simulink model "test_PLECS"  (R2023b)
settings: Solver=VariableStepAuto  StartTime=0.0  StopTime=0.0117  FixedStep=6.5e-6  MaxStep=6.5e-6  MinStep=4.5e-6  RelTol=1e-3
undefined symbols (not defined in the file or in its folder): plecs
libraries: simulink_extras x8
settings Model: Creator=Nelson  LastModifiedBy=franc

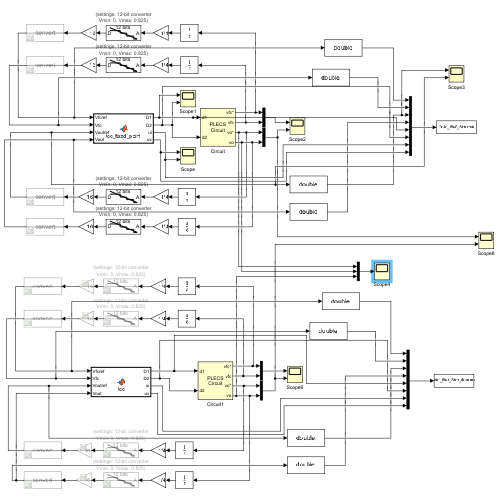
[thumbnail: Simulink's stored preview of the top-level diagram]
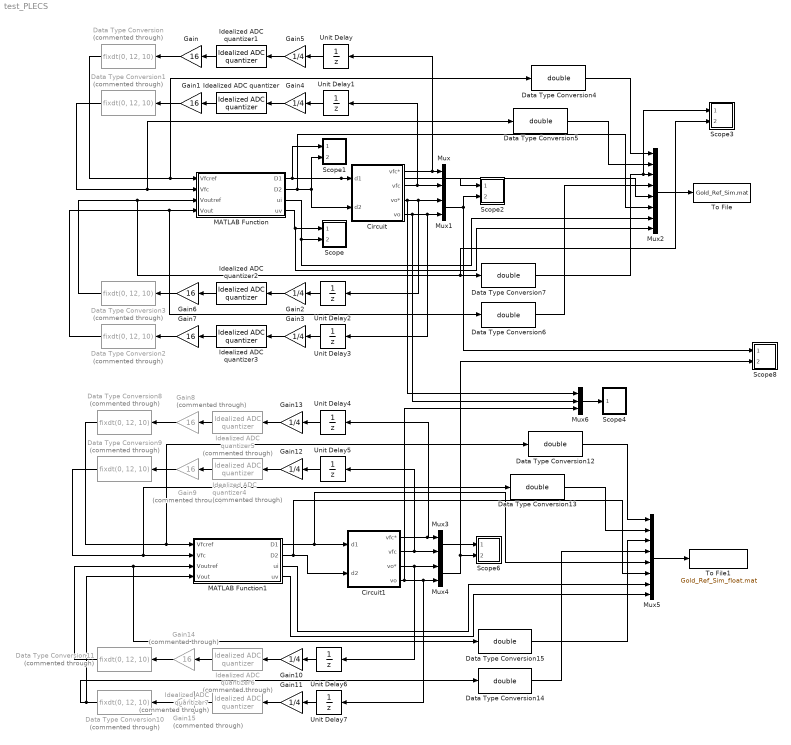
== system test_PLECS ==
  Circuit : Subsystem  LoadFcn=plecs('sl', 200);  InitFcn=plecs('sl', 214);  StartFcn=plecs('sl', 208);  StopFcn=plecs('sl', 209);  mask(PlecsCircuit){PLECSData=<binary blob, 9000 chars, not shown>}
      mask prompts: PLECSData "PLECS Data (Do not delete or modify!)"
      mask init:
      | % PLACE CUSTOM INITIALIZATIONS ABOVE
      | % DO NOT REMOVE
      | plecs('sl', 215);
      | % DO NOT REMOVE
      settings: CopyFcn=plecs('sl', 203);  DeleteFcn=plecs('sl', 205);  UndoDeleteFcn=plecs('sl', 206);  PreSaveFcn=plecs('sl', 211);  PostSaveFcn=plecs('sl', 201);  NameChangeFcn=plecs('sl', 210);  DestroyFcn=plecs('sl', 207);  PreCopyFcn=plecs('sl', 216);  OpenFcn=plecs('sl', 202);  ErrorFcn=plerrorfcn
      mask Help: eval('plecs(''help'', ''qthelp:///creatingacircuit.html'')')
      mask Display: disp('PLECS\nCircuit')
  Circuit1 : Subsystem  LoadFcn=plecs('sl', 200);  InitFcn=plecs('sl', 214);  StartFcn=plecs('sl', 208);  StopFcn=plecs('sl', 209);  mask(PlecsCircuit){PLECSData=<binary blob, 8936 chars, not shown>}
      mask prompts: PLECSData "PLECS Data (Do not delete or modify!)"
      mask init:
      | % PLACE CUSTOM INITIALIZATIONS ABOVE
      | % DO NOT REMOVE
      | plecs('sl', 215);
      | % DO NOT REMOVE
      settings: CopyFcn=plecs('sl', 203);  DeleteFcn=plecs('sl', 205);  UndoDeleteFcn=plecs('sl', 206);  PreSaveFcn=plecs('sl', 211);  PostSaveFcn=plecs('sl', 201);  NameChangeFcn=plecs('sl', 210);  DestroyFcn=plecs('sl', 207);  PreCopyFcn=plecs('sl', 216);  OpenFcn=plecs('sl', 202);  ErrorFcn=plerrorfcn
      mask Help: eval('plecs(''help'', ''qthelp:///creatingacircuit.html'')')
      mask Display: disp('PLECS\nCircuit')
  Data Type Conversion{,1..3,8..11} (8 alike) : DataTypeConversion  Commented=through  OutDataTypeStr=fixdt(0, 12, 10)  RndMeth=Nearest
  Data Type Conversion{4..7,12..15} (8 alike) : DataTypeConversion  OutDataTypeStr=double  RndMeth=Nearest
  Gain{,1,6..7} (4 alike) : Gain  Gain=16  OutDataTypeStr=uint16  RndMeth=Nearest  SaturateOnIntegerOverflow=on
  Gain{2..5,10..13} (8 alike) : Gain  Gain=1/4
  Gain{8..9,14..15} (4 alike) : Gain  Commented=through  Gain=16  OutDataTypeStr=uint16  RndMeth=Nearest  SaturateOnIntegerOverflow=on
  Idealized ADC quantizer{,1..3} (4 alike) : simulink_extras/Additional Discrete/Idealized ADC quantizer  NumberOfConverterBits=12  Vmin=0  Vmax=0.825  OutputDataType=uint16  OutputNegativeValues=off
  Idealized ADC quantizer4 : simulink_extras/Additional Discrete/Idealized ADC quantizer  Commented=through  NumberOfConverterBits=12  Vmin=0  Vmax=0.825  OutputDataType=double  OutputNegativeValues=off
  Idealized ADC quantizer5 : simulink_extras/Additional Discrete/Idealized ADC quantizer  Commented=through  NumberOfConverterBits=12  Vmin=0  Vmax=0.825  OutputDataType=double  OutputNegativeValues=off
  Idealized ADC quantizer6 : simulink_extras/Additional Discrete/Idealized ADC quantizer  Commented=through  NumberOfConverterBits=12  Vmin=0  Vmax=0.825  OutputDataType=uint16  OutputNegativeValues=off
  Idealized ADC quantizer7 : simulink_extras/Additional Discrete/Idealized ADC quantizer  Commented=through  NumberOfConverterBits=12  Vmin=0  Vmax=0.825  OutputDataType=uint16  OutputNegativeValues=off
  MATLAB Function : MATLAB Function  TreatAsAtomicUnit=on
  MATLAB Function1 : MATLAB Function  TreatAsAtomicUnit=on
  Mux{,1,3..4} (4 alike) : Mux  Inputs=2
  Mux2 : Mux  Inputs=8
  Mux5 : Mux  Inputs=8
  Mux6 : Mux  Inputs=3
  Scope : Subsystem  LoadFcn=plecs('sl', 300);  InitFcn=plecs('sl', 314);  StartFcn=plecs('sl', 308);  StopFcn=plecs('sl', 309);  mask{Settings=<binary blob, 900 chars, not shown>}
      mask init:
      | plecs('sl', 315);
      settings: CopyFcn=plecs('sl', 303);  DeleteFcn=plecs('sl', 305);  UndoDeleteFcn=plecs('sl', 306);  PreSaveFcn=plecs('sl', 311);  NameChangeFcn=plecs('sl', 310);  DestroyFcn=plecs('sl', 307);  OpenFcn=plecs('sl', 302);  ErrorFcn=plerrorfcn
      mask Display: plot([0.1 0.9 0.9 0.1 0.1], [0.9 0.9 0.5 0.5 0.9])
  Scope1 : Subsystem  LoadFcn=plecs('sl', 300);  InitFcn=plecs('sl', 314);  StartFcn=plecs('sl', 308);  StopFcn=plecs('sl', 309);  mask{Settings=<binary blob, 888 chars, not shown>}
      mask init:
      | plecs('sl', 315);
      settings: CopyFcn=plecs('sl', 303);  DeleteFcn=plecs('sl', 305);  UndoDeleteFcn=plecs('sl', 306);  PreSaveFcn=plecs('sl', 311);  NameChangeFcn=plecs('sl', 310);  DestroyFcn=plecs('sl', 307);  OpenFcn=plecs('sl', 302);  ErrorFcn=plerrorfcn
      mask Display: plot([0.1 0.9 0.9 0.1 0.1], [0.9 0.9 0.5 0.5 0.9])
  Scope2 : Subsystem  LoadFcn=plecs('sl', 300);  InitFcn=plecs('sl', 314);  StartFcn=plecs('sl', 308);  StopFcn=plecs('sl', 309);  mask{Settings=<binary blob, 1240 chars, not shown>}
      mask init:
      | plecs('sl', 315);
      settings: CopyFcn=plecs('sl', 303);  DeleteFcn=plecs('sl', 305);  UndoDeleteFcn=plecs('sl', 306);  PreSaveFcn=plecs('sl', 311);  NameChangeFcn=plecs('sl', 310);  DestroyFcn=plecs('sl', 307);  OpenFcn=plecs('sl', 302);  ErrorFcn=plerrorfcn
      mask Display: plot([0.1 0.9 0.9 0.1 0.1], [0.9 0.9 0.5 0.5 0.9])
  Scope3 : Subsystem  LoadFcn=plecs('sl', 300);  InitFcn=plecs('sl', 314);  StartFcn=plecs('sl', 308);  StopFcn=plecs('sl', 309);  mask{Settings=<binary blob, 1240 chars, not shown>}
      mask init:
      | plecs('sl', 315);
      settings: CopyFcn=plecs('sl', 303);  DeleteFcn=plecs('sl', 305);  UndoDeleteFcn=plecs('sl', 306);  PreSaveFcn=plecs('sl', 311);  NameChangeFcn=plecs('sl', 310);  DestroyFcn=plecs('sl', 307);  OpenFcn=plecs('sl', 302);  ErrorFcn=plerrorfcn
      mask Display: plot([0.1 0.9 0.9 0.1 0.1], [0.9 0.9 0.5 0.5 0.9])
  Scope4 : Subsystem  LoadFcn=plecs('sl', 300);  InitFcn=plecs('sl', 314);  StartFcn=plecs('sl', 308);  StopFcn=plecs('sl', 309);  mask{Settings=<binary blob, 968 chars, not shown>}
      mask init:
      | plecs('sl', 315);
      settings: CopyFcn=plecs('sl', 303);  DeleteFcn=plecs('sl', 305);  UndoDeleteFcn=plecs('sl', 306);  PreSaveFcn=plecs('sl', 311);  NameChangeFcn=plecs('sl', 310);  DestroyFcn=plecs('sl', 307);  OpenFcn=plecs('sl', 302);  ErrorFcn=plerrorfcn
      mask Display: plot([0.1 0.9 0.9 0.1 0.1], [0.9 0.9 0.5 0.5 0.9])
  Scope6 : Subsystem  LoadFcn=plecs('sl', 300);  InitFcn=plecs('sl', 314);  StartFcn=plecs('sl', 308);  StopFcn=plecs('sl', 309);  mask{Settings=<binary blob, 1240 chars, not shown>}
      mask init:
      | plecs('sl', 315);
      settings: CopyFcn=plecs('sl', 303);  DeleteFcn=plecs('sl', 305);  UndoDeleteFcn=plecs('sl', 306);  PreSaveFcn=plecs('sl', 311);  NameChangeFcn=plecs('sl', 310);  DestroyFcn=plecs('sl', 307);  OpenFcn=plecs('sl', 302);  ErrorFcn=plerrorfcn
      mask Display: plot([0.1 0.9 0.9 0.1 0.1], [0.9 0.9 0.5 0.5 0.9])
  Scope8 : Subsystem  LoadFcn=plecs('sl', 300);  InitFcn=plecs('sl', 314);  StartFcn=plecs('sl', 308);  StopFcn=plecs('sl', 309);  mask{Settings=<binary blob, 1196 chars, not shown>}
      mask init:
      | plecs('sl', 315);
      settings: CopyFcn=plecs('sl', 303);  DeleteFcn=plecs('sl', 305);  UndoDeleteFcn=plecs('sl', 306);  PreSaveFcn=plecs('sl', 311);  NameChangeFcn=plecs('sl', 310);  DestroyFcn=plecs('sl', 307);  OpenFcn=plecs('sl', 302);  ErrorFcn=plerrorfcn
      mask Display: plot([0.1 0.9 0.9 0.1 0.1], [0.9 0.9 0.5 0.5 0.9])
  To File : ToFile  Filename=Gold_Ref_Sim.mat  SampleTime=6.5e-6
  To File1 : ToFile  Filename=Gold_Ref_Sim_float.mat  SampleTime=6.5e-6
  Unit Delay{,1..7} (8 alike) : UnitDelay  SampleTime=-1  HasFrameUpgradeWarning=on
  wires:
  MATLAB Function/2(D2) -> Mux2/6, Scope1/2(2), Circuit/2(d2)
  MATLAB Function/4(uv) -> Mux2/8, Scope/1(1)
  MATLAB Function/3(ui) -> Mux2/7, Scope/2(2)
  Circuit/1(vfc*) -> Unit Delay/1, Mux/1
  Circuit/2(vfc) -> Unit Delay1/1, Mux/2
  Circuit/3(vo*) -> Mux6/1, Unit Delay2/1, Mux1/1
  Circuit/4(vo) -> Mux6/2, Unit Delay3/1, Mux1/2
  Mux/1 -> Scope2/1(1)
  Mux1/1 -> Scope2/2(2), Scope8/1(1)
  Unit Delay2/1 -> Gain2/1
  Idealized ADC quantizer1/1 -> Gain/1
  Gain/1 -> Data Type Conversion/1
  Idealized ADC quantizer/1 -> Gain1/1
  Data Type Conversion/1 -> Data Type Conversion4/1, MATLAB Function/1(Vfcref)
  Gain1/1 -> Data Type Conversion1/1
  Data Type Conversion1/1 -> Data Type Conversion5/1, MATLAB Function/2(Vfc)
  Idealized ADC quantizer3/1 -> Gain7/1
  Idealized ADC quantizer2/1 -> Gain6/1
  Data Type Conversion3/1 -> Scope3/2(2), Data Type Conversion7/1, MATLAB Function/3(Voutref)
  Gain2/1 -> Idealized ADC quantizer2/1
  Unit Delay3/1 -> Gain3/1
  Gain3/1 -> Idealized ADC quantizer3/1
  Gain4/1 -> Idealized ADC quantizer/1
  Unit Delay1/1 -> Gain4/1
  Gain5/1 -> Idealized ADC quantizer1/1
  Unit Delay/1 -> Gain5/1
  Gain6/1 -> Data Type Conversion3/1
  Gain7/1 -> Data Type Conversion2/1
  Mux2/1 -> To File/1
  Data Type Conversion4/1 -> Mux2/1
  Data Type Conversion5/1 -> Mux2/2
  Data Type Conversion2/1 -> Data Type Conversion6/1, MATLAB Function/4(Vout)
  MATLAB Function/1(D1) -> Scope1/1(1), Mux2/5, Circuit/1(d1)
  Data Type Conversion6/1 -> Mux2/4
  Data Type Conversion7/1 -> Scope3/1(1), Mux2/3
  Data Type Conversion13/1 -> Mux5/2
  Gain15/1 -> Data Type Conversion10/1
  Mux5/1 -> To File1/1
  Data Type Conversion12/1 -> Mux5/1
  Unit Delay4/1 -> Gain13/1
  Data Type Conversion14/1 -> Mux5/4
  Gain14/1 -> Data Type Conversion11/1
  Idealized ADC quantizer4/1 -> Gain9/1
  Gain8/1 -> Data Type Conversion8/1
  Circuit1/1(vfc*) -> Unit Delay4/1, Mux3/1
  Data Type Conversion8/1 -> Data Type Conversion12/1, MATLAB Function1/1(Vfcref)
  Idealized ADC quantizer7/1 -> Gain15/1
  Mux4/1 -> Scope6/2(2), Scope8/2(2)
  Circuit1/3(vo*) -> Unit Delay6/1, Mux4/1
  Unit Delay5/1 -> Gain12/1
  Data Type Conversion11/1 -> Data Type Conversion15/1, MATLAB Function1/3(Voutref)
  Unit Delay7/1 -> Gain11/1
  Gain11/1 -> Idealized ADC quantizer7/1
  Gain9/1 -> Data Type Conversion9/1
  Gain13/1 -> Idealized ADC quantizer5/1
  Circuit1/4(vo) -> Mux6/3, Unit Delay7/1, Mux4/2
  Data Type Conversion9/1 -> Data Type Conversion13/1, MATLAB Function1/2(Vfc)
  MATLAB Function1/3(ui) -> Mux5/7
  Data Type Conversion10/1 -> Data Type Conversion14/1, MATLAB Function1/4(Vout)
  MATLAB Function1/1(D1) -> Circuit1/1(d1), Mux5/5
  Circuit1/2(vfc) -> Unit Delay5/1, Mux3/2
  Idealized ADC quantizer6/1 -> Gain14/1
  Gain10/1 -> Idealized ADC quantizer6/1
  MATLAB Function1/4(uv) -> Mux5/8
  MATLAB Function1/2(D2) -> Mux5/6, Circuit1/2(d2)
  Data Type Conversion15/1 -> Mux5/3
  Idealized ADC quantizer5/1 -> Gain8/1
  Unit Delay6/1 -> Gain10/1
  Gain12/1 -> Idealized ADC quantizer4/1
  Mux3/1 -> Scope6/1(1)
  Mux6/1 -> Scope4/1(1)

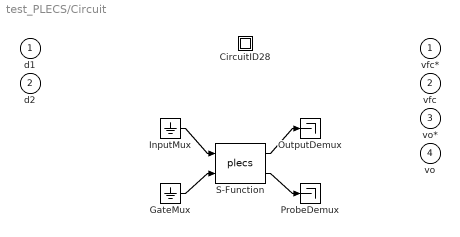
== system test_PLECS/Circuit ==
  d1 : Inport  PortDimensions=1
  d2 : Inport  Port=2  PortDimensions=1
  " CircuitID28 " : Subsystem
  " GateMux " : Ground
  " InputMux " : Ground
  " OutputDemux " : Terminator
  " ProbeDemux " : Terminator
  " S-Function " : S-Function  FunctionName=plecs  SFunctionDeploymentMode=off  EnableBusSupport=off
  vfc* : Outport  PortDimensions=1
  vfc : Outport  Port=2  PortDimensions=1
  vo* : Outport  Port=3  PortDimensions=1
  vo : Outport  Port=4  PortDimensions=1
  wires:
  " InputMux "/1 -> " S-Function "/1
  " GateMux "/1 -> " S-Function "/2
  " S-Function "/1 -> " OutputDemux "/1
  " S-Function "/2 -> " ProbeDemux "/1

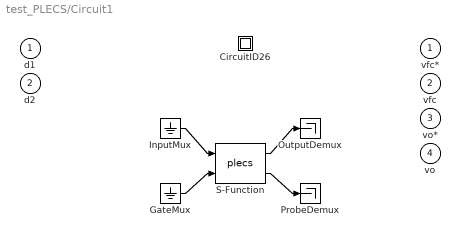
== system test_PLECS/Circuit1 ==
  d1 : Inport  PortDimensions=1
  d2 : Inport  Port=2  PortDimensions=1
  " CircuitID26 " : Subsystem
  " GateMux " : Ground
  " InputMux " : Ground
  " OutputDemux " : Terminator
  " ProbeDemux " : Terminator
  " S-Function " : S-Function  FunctionName=plecs  SFunctionDeploymentMode=off  EnableBusSupport=off
  vfc* : Outport  PortDimensions=1
  vfc : Outport  Port=2  PortDimensions=1
  vo* : Outport  Port=3  PortDimensions=1
  vo : Outport  Port=4  PortDimensions=1
  wires:
  " InputMux "/1 -> " S-Function "/1
  " GateMux "/1 -> " S-Function "/2
  " S-Function "/1 -> " OutputDemux "/1
  " S-Function "/2 -> " ProbeDemux "/1

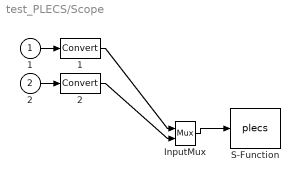
== system test_PLECS/Scope ==
  1 : Inport
  2 : Inport  Port=2
  " 1 " : DataTypeConversion
  " 2 " : DataTypeConversion
  " InputMux " : Mux  Inputs=2
  " S-Function " : S-Function  FunctionName=plecs  SFunctionDeploymentMode=off  EnableBusSupport=off
  wires:
  " InputMux "/1 -> " S-Function "/1
  1/1 -> " 1 "/1
  " 1 "/1 -> " InputMux "/1
  2/1 -> " 2 "/1
  " 2 "/1 -> " InputMux "/2

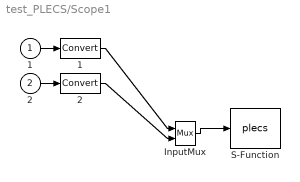
== system test_PLECS/Scope1 ==
  1 : Inport
  2 : Inport  Port=2
  " 1 " : DataTypeConversion
  " 2 " : DataTypeConversion
  " InputMux " : Mux  Inputs=2
  " S-Function " : S-Function  FunctionName=plecs  SFunctionDeploymentMode=off  EnableBusSupport=off
  wires:
  " InputMux "/1 -> " S-Function "/1
  1/1 -> " 1 "/1
  " 1 "/1 -> " InputMux "/1
  2/1 -> " 2 "/1
  " 2 "/1 -> " InputMux "/2

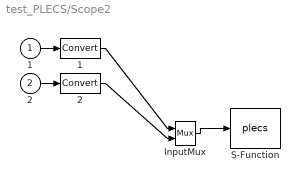
== system test_PLECS/Scope2 ==
  1 : Inport
  2 : Inport  Port=2
  " 1 " : DataTypeConversion
  " 2 " : DataTypeConversion
  " InputMux " : Mux  Inputs=2
  " S-Function " : S-Function  FunctionName=plecs  SFunctionDeploymentMode=off  EnableBusSupport=off
  wires:
  " InputMux "/1 -> " S-Function "/1
  1/1 -> " 1 "/1
  " 1 "/1 -> " InputMux "/1
  2/1 -> " 2 "/1
  " 2 "/1 -> " InputMux "/2

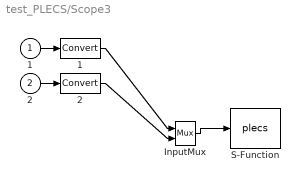
== system test_PLECS/Scope3 ==
  1 : Inport
  2 : Inport  Port=2
  " 1 " : DataTypeConversion
  " 2 " : DataTypeConversion
  " InputMux " : Mux  Inputs=2
  " S-Function " : S-Function  FunctionName=plecs  SFunctionDeploymentMode=off  EnableBusSupport=off
  wires:
  " InputMux "/1 -> " S-Function "/1
  1/1 -> " 1 "/1
  " 1 "/1 -> " InputMux "/1
  2/1 -> " 2 "/1
  " 2 "/1 -> " InputMux "/2

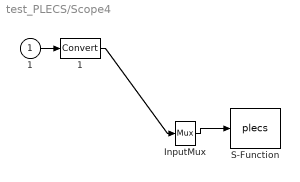
== system test_PLECS/Scope4 ==
  1 : Inport
  " 1 " : DataTypeConversion
  " InputMux " : Mux  Inputs=1
  " S-Function " : S-Function  FunctionName=plecs  SFunctionDeploymentMode=off  EnableBusSupport=off
  wires:
  " InputMux "/1 -> " S-Function "/1
  1/1 -> " 1 "/1
  " 1 "/1 -> " InputMux "/1

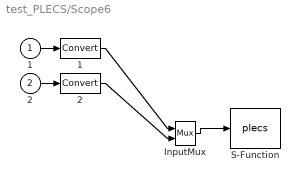
== system test_PLECS/Scope6 ==
  1 : Inport
  2 : Inport  Port=2
  " 1 " : DataTypeConversion
  " 2 " : DataTypeConversion
  " InputMux " : Mux  Inputs=2
  " S-Function " : S-Function  FunctionName=plecs  SFunctionDeploymentMode=off  EnableBusSupport=off
  wires:
  " InputMux "/1 -> " S-Function "/1
  1/1 -> " 1 "/1
  " 1 "/1 -> " InputMux "/1
  2/1 -> " 2 "/1
  " 2 "/1 -> " InputMux "/2

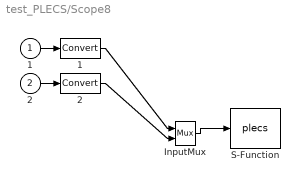
== system test_PLECS/Scope8 ==
  1 : Inport
  2 : Inport  Port=2
  " 1 " : DataTypeConversion
  " 2 " : DataTypeConversion
  " InputMux " : Mux  Inputs=2
  " S-Function " : S-Function  FunctionName=plecs  SFunctionDeploymentMode=off  EnableBusSupport=off
  wires:
  " InputMux "/1 -> " S-Function "/1
  1/1 -> " 1 "/1
  " 1 "/1 -> " InputMux "/1
  2/1 -> " 2 "/1
  " 2 "/1 -> " InputMux "/2

== system test_PLECS/Circuit/ CircuitID28  ==

== system test_PLECS/Circuit1/ CircuitID26  ==

== matlab function test_PLECS/MATLAB Function1 ==
  data: Vfcref input; Vfc input; Voutref input; Vout input; D1 output; D2 output; ui output; uv output
function [D1, D2, ui, uv] = fcc(Vfcref, Vfc, Voutref, Vout)
    % Kpv =  3.214624;
    % Kiv = -1.410335;
    % Kpc =  12.58407884;
    % Kic = -12.410690825;
    % MAX_DUTY_CYCLE = (127);
    % gain = 4/65535;
    % 
    % ui_aux = pivo_fun(Voutref*gain, Vout*gain, 0.0, 127.0, Kpv, Kiv);
    % uv_aux = pivf_fun(Vfcref*gain , Vfc*gain , -38.0, 38.0, Kpc, Kic);

    Kpv = 0.025312;
    Kiv = -0.011105;
    Kpc =  0.099087235;
    Kic = -0.097721975;
    MAX_DUTY_CYCLE = (127);
    gain = 4;

    ui_aux = pivo_fun(Voutref*gain, Vout*gain, 0.0, 1.0, Kpv, Kiv);
    uv_aux = pivf_fun(Vfcref*gain , Vfc*gain , -0.3, 0.3, Kpc, Kic);


    D1_aux = ((ui_aux) + (uv_aux))*MAX_DUTY_CYCLE;
    D2_aux = ((ui_aux) - (uv_aux))*MAX_DUTY_CYCLE;

    D1  = max(0, min(D1_aux, MAX_DUTY_CYCLE));
    D2  = max(0, min(D2_aux, MAX_DUTY_CYCLE));

    ui = (ui_aux);
    uv = (uv_aux);
end

%function out = pivf_fun(varargin)
function out = pivf_fun(Vrk, Vk, Vmin, Vmax, Kpid, Kiid)
    % Declarar todas las variables persistentes al inicio
    persistent Kp Ki KUi KXi
    persistent xVrk xVk xVmax xVmin xXik xUik xVmk

    % Inicializar si es primera vez
    if isempty(xXik)
        xXik = zeros(1, 2);
        xUik = zeros(1, 2);
    end

    % Asignación de parámetros
    xVrk = Vrk;
    xVk = Vk;
    xVmax = Vmax;
    xVmin = Vmin;
    Kp = Kpid;
    Ki = Kiid;
    KUi = -(Kp + Ki)/(Kp * Kpid);
    KXi = -Ki / Kp;

    % PI cálculo
    xXik(2) = xXik(1);
    xUik(2) = xUik(1);
    xXik(1) = KUi * xUik(2) + KXi * xXik(2);
    xUik(1) = Kp * (xVrk - xVk - xXik(1));
    xUik(1) = min(max(xUik(1), xVmin), xVmax);

    xVmk = xUik(1);
    out = xVmk;
end

%function out = pivf_fun(varargin)
function out = pivo_fun(Vrk, Vk, Vmin, Vmax, Kpid, Kiid)
    % Declarar todas las variables persistentes al inicio
    persistent Kp Ki KUi KXi
    persistent xVrk xVk xVmax xVmin xXik xUik xVmk

    % Inicializar si es primera vez
    if isempty(xXik)
        xXik = zeros(1, 2);
        xUik = zeros(1, 2);
    end

    % Asignación de parámetros
    xVrk = Vrk;
    xVk = Vk;
    xVmax = Vmax;
    xVmin = Vmin;
    Kp = Kpid;
    Ki = Kiid;
    KUi = -(Kp + Ki)/(Kp * Kpid);
    KXi = -Ki / Kp;

    % PI cálculo
    xXik(2) = xXik(1);
    xUik(2) = xUik(1);
    xXik(1) = KUi * xUik(2) + KXi * xXik(2);
    xUik(1) = Kp * (xVrk - xVk - xXik(1));
    xUik(1) = min(max(xUik(1), xVmin), xVmax);

    xVmk = xUik(1);
    out = xVmk;
end

== matlab function test_PLECS/MATLAB Function ==
  data: Vfcref input; Vfc input; Voutref input; Vout input; D1 output; D2 output; ui output; uv output
%%%%%%%%%%%%%%%%%%%%%%%%%%%%%%%%%%%%%%%%%%%%%%%%%%%%%%%%%%%%%%%%%%%%%%%%%%%%
%                                                                          %
%          Generated by MATLAB 23.2 and Fixed-Point Designer 23.2          %
%                                                                          %
%%%%%%%%%%%%%%%%%%%%%%%%%%%%%%%%%%%%%%%%%%%%%%%%%%%%%%%%%%%%%%%%%%%%%%%%%%%%
function [D1,D2,ui,uv] = fcc_fixed_point(Vfcref,Vfc,Voutref,Vout)
    fm = get_fimath();
    Vfcref_in = fi( Vfcref, 0, 16, 0, fm );
    Vfc_in = fi( Vfc, 0, 16, 0, fm );
    Voutref_in = fi( Voutref, 0, 16, 0, fm );
    Vout_in = fi( Vout, 0, 16, 0, fm );
    [D1_out,D2_out,ui_out,uv_out] = fcc_fixpt( Vfcref_in, Vfc_in, Voutref_in, Vout_in );
    D1 = double( D1_out );
    D2 = double( D2_out );
    ui = double( ui_out );
    uv = double( uv_out );
end

function [D1, D2, ui, uv] = fcc_fixpt(Vfcref, Vfc, Voutref, Vout)
    fm = get_fimath();

    Kpv =  fi(3.214624, 1, 22, 14, fm);
    Kiv = fi(-1.4105, 1, 22, 14, fm);fi(335, 0, 9, 0, fm);
    Kpc =  fi(12.58407884, 1, 22, 14, fm);
    Kic = fi(-12.410690825, 1, 22, 14, fm);
    MAX_DUTY_CYCLE = fi((127), 0, 8, 0, fm);
    gain = fi(4/65535, 1, 22, 14, fm);
    %D1_aux = int8(0);
    %D2_aux = int8(0);

    % Calculo de actuaciones desacopladas
    %ui_aux = int8(0);
    %uv_aux = int8(0);
    ui_aux = fi(pivo_fun(fi(Voutref*gain, 1, 22, 14, fm), fi(Vout*gain, 1, 22, 14, fm), fi(fi(0.0, 0, 1, 0, fm), 1, 22, 14, fm), fi(fi(127.0, 0, 7, 0, fm), 1, 22, 14, fm), fi(Kpv, 1, 22, 14, fm), fi(Kiv, 1, 22, 14, fm)), 1, 22, 14, fm);
    uv_aux = fi(pivf_fun(fi(Vfcref*gain, 1, 22, 14, fm) , fi(Vfc*gain, 1, 22, 14, fm) , fi(fi(-38.0, 1, 7, 0, fm), 1, 22, 14, fm), fi(fi(38.0, 0, 6, 0, fm), 1, 22, 14, fm), fi(Kpc, 1, 22, 14, fm), fi(Kic, 1, 22, 14, fm)), 1, 22, 14, fm);


    D1_aux = fi(fix((ui_aux) + (uv_aux)), 0, 8, 0, fm);
    D2_aux = fi(fix((ui_aux) - (uv_aux)), 0, 8, 0, fm);

    D1 = fi((min(D1_aux, MAX_DUTY_CYCLE)), 0, 8, 0, fm);
    D2 = fi((min(D2_aux, MAX_DUTY_CYCLE)), 0, 8, 0, fm);

    ui = fi((ui_aux), 0, 8, 0, fm);
    uv = fi((uv_aux), 0, 8, 0, fm);
end

%function out = pivf_fun(varargin)
function out = pivo_fun(Vrk, Vk, Vmin, Vmax, Kpid, Kiid)
    % Declarar todas las variables persistentes al inicio
    fm = get_fimath();

    persistent Kp Ki KUi KXi
    persistent xVrk xVk xVmax xVmin xXik xUik xVmk

    % --------------------------
    % Caso: RESET con un solo argumento
    % --------------------------
    %if nargin == 1 && islogical(varargin{1}) && varargin{1} == true
    %    clear pivo_fun
    %    out = 0.0;
    %    return
    %end

    % --------------------------
    % Caso: operación normal
    % --------------------------
    %if nargin ~= 7
    %    error('pivo_fun: Expected 7 input arguments or reset flag.');
    %end

    % Extraer argumentos normalmente
    %Vrk  = varargin{1};
    %Vk   = varargin{2};
    %Vmin = varargin{3};
    %Vmax = varargin{4};
    %Kpid = varargin{5};
    %Kiid = varargin{6};
    %reset = varargin{7}; %#ok<NASGU>  % No se usa ya

    % Inicializar si es primera vez
    if isempty(xXik)
        xXik = fi(zeros(1, 2), 1, 22, 14, fm);
        xUik = fi(zeros(1, 2), 1, 22, 14, fm);
    end

    % Asignación de parámetros
    xVrk = fi(Vrk, 1, 22, 14, fm);
    xVk = fi(Vk, 1, 22, 14, fm);
    xVmax = fi(Vmax, 1, 22, 14, fm);
    xVmin = fi(Vmin, 1, 22, 14, fm);
    Kp = fi(Kpid, 1, 22, 14, fm);
    Ki = fi(Kiid, 1, 22, 14, fm);
    KUi = fi(fi_div(fi_uminus((Kp + Ki)), (Kp * Kpid)), 1, 22, 14, fm);
    KXi = fi(fi_div(fi_uminus(Ki), Kp), 1, 22, 14, fm);

    % PI cálculo
    xXik(2) = xXik(1);
    xUik(2) = xUik(1);
    xXik(1) = KUi * xUik(2) + KXi * xXik(2);
    xUik(1) = Kp * (xVrk - xVk - xXik(1));
    xUik(1) = min(max(xUik(1), xVmin), xVmax);

    xVmk = fi(xUik(1), 1, 22, 14, fm);
    out = fi(xVmk, 1, 22, 14, fm);
end

%function out = pivf_fun(varargin)
function out = pivf_fun(Vrk, Vk, Vmin, Vmax, Kpid, Kiid)
    % Declarar todas las variables persistentes al inicio
    fm = get_fimath();

    persistent Kp Ki KUi KXi
    persistent xVrk xVk xVmax xVmin xXik xUik xVmk

    % --------------------------
    % Caso: RESET con un solo argumento
    % --------------------------
    %if nargin == 1 && islogical(varargin{1}) && varargin{1} == true
    %    clear pivo_fun
    %    out = 0.0;
    %    return
    %end

    % --------------------------
    % Caso: operación normal
    % --------------------------
    %if nargin ~= 7
    %    error('pivo_fun: Expected 7 input arguments or reset flag.');
    %end

    % Extraer argumentos normalmente
    %Vrk  = varargin{1};
    %Vk   = varargin{2};
    %Vmin = varargin{3};
    %Vmax = varargin{4};
    %Kpid = varargin{5};
    %Kiid = varargin{6};
    %reset = varargin{7}; %#ok<NASGU>  % No se usa ya

    % Inicializar si es primera vez
    if isempty(xXik)
        xXik = fi(zeros(1, 2), 1, 22, 14, fm);
        xUik = fi(zeros(1, 2), 1, 22, 14, fm);
    end

    % Asignación de parámetros
    xVrk = fi(Vrk, 1, 22, 14, fm);
    xVk = fi(Vk, 1, 22, 14, fm);
    xVmax = fi(Vmax, 1, 22, 14, fm);
    xVmin = fi(Vmin, 1, 22, 14, fm);
    Kp = fi(Kpid, 1, 22, 14, fm);
    Ki = fi(Kiid, 1, 22, 14, fm);
    KUi = fi(fi_div(fi_uminus((Kp + Ki)), (Kp * Kpid)), 1, 22, 14, fm);
    KXi = fi(fi_div(fi_uminus(Ki), Kp), 1, 22, 14, fm);

    % PI cálculo
    xXik(2) = xXik(1);
    xUik(2) = xUik(1);
    xXik(1) = KUi * xUik(2) + KXi * xXik(2);
    xUik(1) = Kp * (fi_signed(xVrk - xVk) - xXik(1));
    xUik(1) = min(max(xUik(1), xVmin), xVmax);

    xVmk = fi(xUik(1), 1, 22, 14, fm);
    out = fi(xVmk, 1, 22, 14, fm);
end



function ntype = divideType(a,b)
    coder.inline( 'always' );
    nt1 = numerictype( a );
    nt2 = numerictype( b );
    maxFL = max( [ min( nt1.WordLength, nt1.FractionLength ), min( nt2.WordLength, nt2.FractionLength ) ] );
    FL = max( maxFL, 24 );
    extraBits = (FL - maxFL);
    WL = nt1.WordLength + nt2.WordLength;
    WL = min( WL, 124 );
    if (WL + extraBits)<64
        ntype = numerictype( nt1.Signed || nt2.Signed, WL + extraBits, FL );
    else
        ntype = numerictype( nt1.Signed || nt2.Signed, WL, FL );
    end
end


function c = fi_div(a,b)
    coder.inline( 'always' );
    a1 = fi( a, 'RoundMode', 'fix' );
    b1 = fi( b, 'RoundMode', 'fix' );
    nType = divideType( a1, b1 );
    if isfi( a ) && isfi( b ) && isscalar( b )
        c1 = divide( nType, a1, b1 );
        c = fi( c1, numerictype( c1 ), fimath( a ) );
    else
        c = fi( a / b, nType );
    end
end


function y = fi_signed(a)
    coder.inline( 'always' );
    if isfi( a ) && ~(issigned( a ))
        nt = numerictype( a );
        new_nt = numerictype( 1, nt.WordLength + 1, nt.FractionLength );
        y = fi( a, new_nt, fimath( a ) );
    else
        y = a;
    end
end


function y = fi_uminus(a)
    coder.inline( 'always' );
    if isfi( a )
        nt = numerictype( a );
        new_nt = numerictype( 1, nt.WordLength + 1, nt.FractionLength );
        y = -fi( a, new_nt, fimath( a ) );
    else
        y = -a;
    end
end

function fm = get_fimath()
	fm = fimath('RoundingMethod', 'Round',...
	     'OverflowAction', 'Saturate',...
	     'ProductMode','FullPrecision',...
	     'SumMode','FullPrecision');
end
